simulink library "BechamoNasaOpenModels"  (R2024a)
settings: Solver=VariableStepAuto  StartTime=0.0  StopTime=10.0  RelTol=1e-3
values from neighbouring files (symbols this model uses):
  Cl_aileron_wing_1 = Cl_mat.Claileron_wing.axes1.value    [setupMavrik.m]
  Cl_aileron_wing_2 = Cl_mat.Claileron_wing.axes2.value    [setupMavrik.m]
  Cl_aileron_wing_3 = Cl_mat.Claileron_wing.axes3.value    [setupMavrik.m]
  Cl_aileron_wing_val = Cl_mat.Claileron_wing.value    [setupMavrik.m]
  Cl_elevator_tail_1 = Cl_mat.Clelevator_tail.axes1.value    [setupMavrik.m]
  Cl_elevator_tail_2 = Cl_mat.Clelevator_tail.axes2.value    [setupMavrik.m]
  Cl_elevator_tail_3 = Cl_mat.Clelevator_tail.axes3.value    [setupMavrik.m]
  Cl_elevator_tail_val = Cl_mat.Clelevator_tail.value    [setupMavrik.m]
  Cl_flap_wing_1 = Cl_mat.Clflap_wing.axes1.value    [setupMavrik.m]
  Cl_flap_wing_2 = Cl_mat.Clflap_wing.axes2.value    [setupMavrik.m]
  Cl_flap_wing_3 = Cl_mat.Clflap_wing.axes3.value    [setupMavrik.m]
  Cl_flap_wing_val = Cl_mat.Clflap_wing.value    [setupMavrik.m]
  Cl_hover_fuse_1 = Cl_mat.Clhover_fuse.axes1.value    [setupMavrik.m]
  Cl_hover_fuse_2 = Cl_mat.Clhover_fuse.axes2.value    [setupMavrik.m]
  Cl_hover_fuse_3 = Cl_mat.Clhover_fuse.axes3.value    [setupMavrik.m]
  Cl_hover_fuse_val = Cl_mat.Clhover_fuse.value    [setupMavrik.m]
  Cl_rudder_tail_1 = Cl_mat.Clrudder_tail.axes1.value    [setupMavrik.m]
  Cl_rudder_tail_2 = Cl_mat.Clrudder_tail.axes2.value    [setupMavrik.m]
  Cl_rudder_tail_3 = Cl_mat.Clrudder_tail.axes3.value    [setupMavrik.m]
  Cl_rudder_tail_val = Cl_mat.Clrudder_tail.value    [setupMavrik.m]
  Cl_tail_1 = Cl_mat.Cltail.axes1.value    [setupMavrik.m]
  Cl_tail_2 = Cl_mat.Cltail.axes2.value    [setupMavrik.m]
  Cl_tail_3 = Cl_mat.Cltail.axes3.value    [setupMavrik.m]
  Cl_tail_damp_p_1 = Cl_mat.Cltail_damp_p.axes1.value    [setupMavrik.m]
  Cl_tail_damp_p_2 = Cl_mat.Cltail_damp_p.axes2.value    [setupMavrik.m]
  Cl_tail_damp_p_3 = Cl_mat.Cltail_damp_p.axes3.value    [setupMavrik.m]
  Cl_tail_damp_p_val = Cl_mat.Cltail_damp_p.value    [setupMavrik.m]
  Cl_tail_damp_q_1 = Cl_mat.Cltail_damp_q.axes1.value    [setupMavrik.m]
  Cl_tail_damp_q_2 = Cl_mat.Cltail_damp_q.axes2.value    [setupMavrik.m]
  Cl_tail_damp_q_3 = Cl_mat.Cltail_damp_q.axes3.value    [setupMavrik.m]
  Cl_tail_damp_q_val = Cl_mat.Cltail_damp_q.value    [setupMavrik.m]
  Cl_tail_damp_r_1 = Cl_mat.Cltail_damp_r.axes1.value    [setupMavrik.m]
  Cl_tail_damp_r_2 = Cl_mat.Cltail_damp_r.axes2.value    [setupMavrik.m]
  Cl_tail_damp_r_3 = Cl_mat.Cltail_damp_r.axes3.value    [setupMavrik.m]
  Cl_tail_damp_r_val = Cl_mat.Cltail_damp_r.value    [setupMavrik.m]
  Cl_tail_val = Cl_mat.Cltail.value    [setupMavrik.m]
  Cl_wing_1 = Cl_mat.Clwing.axes1.value    [setupMavrik.m]
  Cl_wing_2 = Cl_mat.Clwing.axes2.value    [setupMavrik.m]
  Cl_wing_3 = Cl_mat.Clwing.axes3.value    [setupMavrik.m]
  Cl_wing_damp_p_1 = Cl_mat.Clwing_damp_p.axes1.value    [setupMavrik.m]
  Cl_wing_damp_p_2 = Cl_mat.Clwing_damp_p.axes2.value    [setupMavrik.m]
  Cl_wing_damp_p_3 = Cl_mat.Clwing_damp_p.axes3.value    [setupMavrik.m]
  Cl_wing_damp_p_val = Cl_mat.Clwing_damp_p.value    [setupMavrik.m]
  Cl_wing_damp_q_1 = Cl_mat.Clwing_damp_q.axes1.value    [setupMavrik.m]
  Cl_wing_damp_q_2 = Cl_mat.Clwing_damp_q.axes2.value    [setupMavrik.m]
  Cl_wing_damp_q_3 = Cl_mat.Clwing_damp_q.axes3.value    [setupMavrik.m]
  Cl_wing_damp_q_val = Cl_mat.Clwing_damp_q.value    [setupMavrik.m]
  Cl_wing_damp_r_1 = Cl_mat.Clwing_damp_r.axes1.value    [setupMavrik.m]
  Cl_wing_damp_r_2 = Cl_mat.Clwing_damp_r.axes2.value    [setupMavrik.m]
  Cl_wing_damp_r_3 = Cl_mat.Clwing_damp_r.axes3.value    [setupMavrik.m]
  Cl_wing_damp_r_val = Cl_mat.Clwing_damp_r.value    [setupMavrik.m]
  Cl_wing_val = Cl_mat.Clwing.value    [setupMavrik.m]
  Cm_aileron_wing_1 = Cm_mat.Cmaileron_wing.axes1.value    [setupMavrik.m]
  Cm_aileron_wing_2 = Cm_mat.Cmaileron_wing.axes2.value    [setupMavrik.m]
  Cm_aileron_wing_3 = Cm_mat.Cmaileron_wing.axes3.value    [setupMavrik.m]
  Cm_aileron_wing_val = Cm_mat.Cmaileron_wing.value    [setupMavrik.m]
  Cm_elevator_tail_1 = Cm_mat.Cmelevator_tail.axes1.value    [setupMavrik.m]
  Cm_elevator_tail_2 = Cm_mat.Cmelevator_tail.axes2.value    [setupMavrik.m]
  Cm_elevator_tail_3 = Cm_mat.Cmelevator_tail.axes3.value    [setupMavrik.m]
  Cm_elevator_tail_val = Cm_mat.Cmelevator_tail.value    [setupMavrik.m]
  Cm_flap_wing_1 = Cm_mat.Cmflap_wing.axes1.value    [setupMavrik.m]
  Cm_flap_wing_2 = Cm_mat.Cmflap_wing.axes2.value    [setupMavrik.m]
  Cm_flap_wing_3 = Cm_mat.Cmflap_wing.axes3.value    [setupMavrik.m]
  Cm_flap_wing_val = Cm_mat.Cmflap_wing.value    [setupMavrik.m]
  Cm_hover_fuse_1 = Cm_mat.Cmhover_fuse.axes1.value    [setupMavrik.m]
  Cm_hover_fuse_2 = Cm_mat.Cmhover_fuse.axes2.value    [setupMavrik.m]
  Cm_hover_fuse_3 = Cm_mat.Cmhover_fuse.axes3.value    [setupMavrik.m]
  Cm_hover_fuse_val = Cm_mat.Cmhover_fuse.value    [setupMavrik.m]
  Cm_rudder_tail_1 = Cm_mat.Cmrudder_tail.axes1.value    [setupMavrik.m]
  Cm_rudder_tail_2 = Cm_mat.Cmrudder_tail.axes2.value    [setupMavrik.m]
  Cm_rudder_tail_3 = Cm_mat.Cmrudder_tail.axes3.value    [setupMavrik.m]
  Cm_rudder_tail_val = Cm_mat.Cmrudder_tail.value    [setupMavrik.m]
  Cm_tail_1 = Cm_mat.Cmtail.axes1.value    [setupMavrik.m]
  Cm_tail_2 = Cm_mat.Cmtail.axes2.value    [setupMavrik.m]
  Cm_tail_3 = Cm_mat.Cmtail.axes3.value    [setupMavrik.m]
  Cm_tail_damp_p_1 = Cm_mat.Cmtail_damp_p.axes1.value    [setupMavrik.m]
  Cm_tail_damp_p_2 = Cm_mat.Cmtail_damp_p.axes2.value    [setupMavrik.m]
  Cm_tail_damp_p_3 = Cm_mat.Cmtail_damp_p.axes3.value    [setupMavrik.m]
  Cm_tail_damp_p_val = Cm_mat.Cmtail_damp_p.value    [setupMavrik.m]
  Cm_tail_damp_q_1 = Cm_mat.Cmtail_damp_q.axes1.value    [setupMavrik.m]
  Cm_tail_damp_q_2 = Cm_mat.Cmtail_damp_q.axes2.value    [setupMavrik.m]
  Cm_tail_damp_q_3 = Cm_mat.Cmtail_damp_q.axes3.value    [setupMavrik.m]
  Cm_tail_damp_q_val = Cm_mat.Cmtail_damp_q.value    [setupMavrik.m]
  Cm_tail_damp_r_1 = Cm_mat.Cmtail_damp_r.axes1.value    [setupMavrik.m]
  Cm_tail_damp_r_2 = Cm_mat.Cmtail_damp_r.axes2.value    [setupMavrik.m]
  Cm_tail_damp_r_3 = Cm_mat.Cmtail_damp_r.axes3.value    [setupMavrik.m]
  Cm_tail_damp_r_val = Cm_mat.Cmtail_damp_r.value    [setupMavrik.m]
  Cm_tail_val = Cm_mat.Cmtail.value    [setupMavrik.m]
  Cm_wing_1 = Cm_mat.Cmwing.axes1.value    [setupMavrik.m]
  Cm_wing_2 = Cm_mat.Cmwing.axes2.value    [setupMavrik.m]
  Cm_wing_3 = Cm_mat.Cmwing.axes3.value    [setupMavrik.m]
  Cm_wing_damp_p_1 = Cm_mat.Cmwing_damp_p.axes1.value    [setupMavrik.m]
  Cm_wing_damp_p_2 = Cm_mat.Cmwing_damp_p.axes2.value    [setupMavrik.m]
  Cm_wing_damp_p_3 = Cm_mat.Cmwing_damp_p.axes3.value    [setupMavrik.m]
  Cm_wing_damp_p_val = Cm_mat.Cmwing_damp_p.value    [setupMavrik.m]
  Cm_wing_damp_q_1 = Cm_mat.Cmwing_damp_q.axes1.value    [setupMavrik.m]
  Cm_wing_damp_q_2 = Cm_mat.Cmwing_damp_q.axes2.value    [setupMavrik.m]
  Cm_wing_damp_q_3 = Cm_mat.Cmwing_damp_q.axes3.value    [setupMavrik.m]
  Cm_wing_damp_q_val = Cm_mat.Cmwing_damp_q.value    [setupMavrik.m]
  Cm_wing_damp_r_1 = Cm_mat.Cmwing_damp_r.axes1.value    [setupMavrik.m]
  Cm_wing_damp_r_2 = Cm_mat.Cmwing_damp_r.axes2.value    [setupMavrik.m]
  Cm_wing_damp_r_3 = Cm_mat.Cmwing_damp_r.axes3.value    [setupMavrik.m]
  Cm_wing_damp_r_val = Cm_mat.Cmwing_damp_r.value    [setupMavrik.m]
  Cm_wing_val = Cm_mat.Cmwing.value    [setupMavrik.m]
  Cn_aileron_wing_1 = Cn_mat.Cnaileron_wing.axes1.value    [setupMavrik.m]
  Cn_aileron_wing_2 = Cn_mat.Cnaileron_wing.axes2.value    [setupMavrik.m]
  Cn_aileron_wing_3 = Cn_mat.Cnaileron_wing.axes3.value    [setupMavrik.m]
  Cn_aileron_wing_val = Cn_mat.Cnaileron_wing.value    [setupMavrik.m]
  Cn_elevator_tail_1 = Cn_mat.Cnelevator_tail.axes1.value    [setupMavrik.m]
  Cn_elevator_tail_2 = Cn_mat.Cnelevator_tail.axes2.value    [setupMavrik.m]
  Cn_elevator_tail_3 = Cn_mat.Cnelevator_tail.axes3.value    [setupMavrik.m]
  Cn_elevator_tail_val = Cn_mat.Cnelevator_tail.value    [setupMavrik.m]
  Cn_flap_wing_1 = Cn_mat.Cnflap_wing.axes1.value    [setupMavrik.m]
  Cn_flap_wing_2 = Cn_mat.Cnflap_wing.axes2.value    [setupMavrik.m]
  Cn_flap_wing_3 = Cn_mat.Cnflap_wing.axes3.value    [setupMavrik.m]
  Cn_flap_wing_val = Cn_mat.Cnflap_wing.value    [setupMavrik.m]
  Cn_hover_fuse_1 = Cn_mat.Cnhover_fuse.axes1.value    [setupMavrik.m]
  Cn_hover_fuse_2 = Cn_mat.Cnhover_fuse.axes2.value    [setupMavrik.m]
  Cn_hover_fuse_3 = Cn_mat.Cnhover_fuse.axes3.value    [setupMavrik.m]
  Cn_hover_fuse_val = Cn_mat.Cnhover_fuse.value    [setupMavrik.m]
  ... (+318 more)
libraries: matrix_library x15, shared6dof x1, sharedtransform x1
(part 3 of 19)

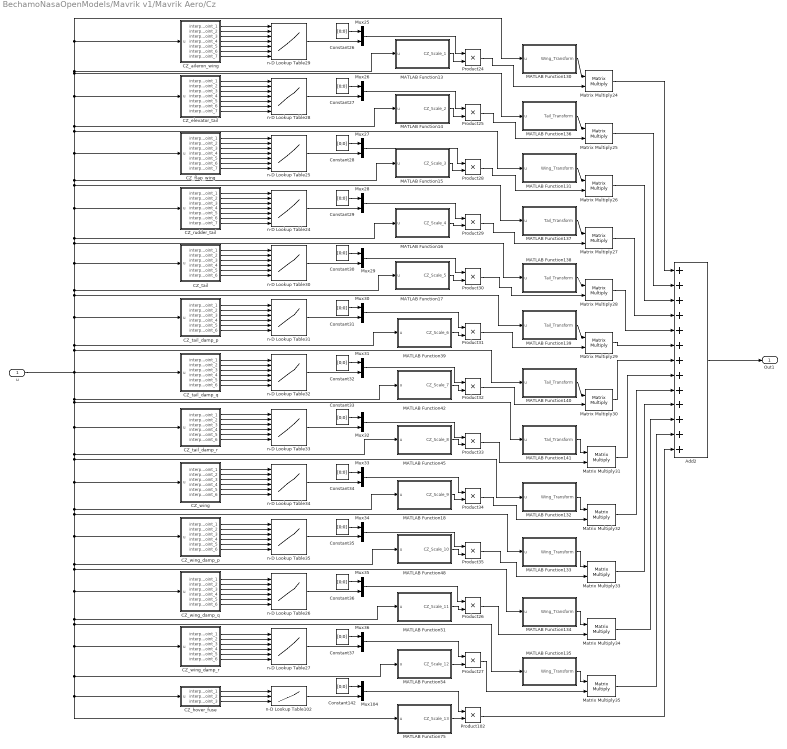
== system BechamoNasaOpenModels/Mavrik v1/Mavrik Aero/Cz ==
  u : Inport
  Add2 : Sum  Inputs=+++++++++++++
  CZ_aileron_wing : MATLAB Function  TreatAsAtomicUnit=on
  CZ_elevator_tail : MATLAB Function  TreatAsAtomicUnit=on
  CZ_flap_wing : MATLAB Function  TreatAsAtomicUnit=on
  CZ_hover_fuse : MATLAB Function  TreatAsAtomicUnit=on
  CZ_rudder_tail : MATLAB Function  TreatAsAtomicUnit=on
  CZ_tail : MATLAB Function  TreatAsAtomicUnit=on
  CZ_tail_damp_p : MATLAB Function  TreatAsAtomicUnit=on
  CZ_tail_damp_q : MATLAB Function  TreatAsAtomicUnit=on
  CZ_tail_damp_r : MATLAB Function  TreatAsAtomicUnit=on
  CZ_wing : MATLAB Function  TreatAsAtomicUnit=on
  CZ_wing_damp_p : MATLAB Function  TreatAsAtomicUnit=on
  CZ_wing_damp_q : MATLAB Function  TreatAsAtomicUnit=on
  CZ_wing_damp_r : MATLAB Function  TreatAsAtomicUnit=on
  Constant{26..37,142} (13 alike) : Constant  Value=[0;0]
  MATLAB Function13 : MATLAB Function  TreatAsAtomicUnit=on
  MATLAB Function130 : MATLAB Function  TreatAsAtomicUnit=on
  MATLAB Function131 : MATLAB Function  TreatAsAtomicUnit=on
  MATLAB Function132 : MATLAB Function  TreatAsAtomicUnit=on
  MATLAB Function133 : MATLAB Function  TreatAsAtomicUnit=on
  MATLAB Function134 : MATLAB Function  TreatAsAtomicUnit=on
  MATLAB Function135 : MATLAB Function  TreatAsAtomicUnit=on
  MATLAB Function136 : MATLAB Function  TreatAsAtomicUnit=on
  MATLAB Function137 : MATLAB Function  TreatAsAtomicUnit=on
  MATLAB Function138 : MATLAB Function  TreatAsAtomicUnit=on
  MATLAB Function139 : MATLAB Function  TreatAsAtomicUnit=on
  MATLAB Function14 : MATLAB Function  TreatAsAtomicUnit=on
  MATLAB Function140 : MATLAB Function  TreatAsAtomicUnit=on
  MATLAB Function141 : MATLAB Function  TreatAsAtomicUnit=on
  MATLAB Function15 : MATLAB Function  TreatAsAtomicUnit=on
  MATLAB Function16 : MATLAB Function  TreatAsAtomicUnit=on
  MATLAB Function17 : MATLAB Function  TreatAsAtomicUnit=on
  MATLAB Function18 : MATLAB Function  TreatAsAtomicUnit=on
  MATLAB Function39 : MATLAB Function  TreatAsAtomicUnit=on
  MATLAB Function42 : MATLAB Function  TreatAsAtomicUnit=on
  MATLAB Function45 : MATLAB Function  TreatAsAtomicUnit=on
  MATLAB Function48 : MATLAB Function  TreatAsAtomicUnit=on
  MATLAB Function51 : MATLAB Function  TreatAsAtomicUnit=on
  MATLAB Function54 : MATLAB Function  TreatAsAtomicUnit=on
  MATLAB Function75 : MATLAB Function  TreatAsAtomicUnit=on
  Matrix Multiply{24..35} (12 alike) : Product  Multiplication=Matrix(*)
  Mux{25..36,104} (13 alike) : Mux  Inputs=2
  Product{24..35,102} (13 alike) : Product
  n-D Lookup Table102 : Lookup_n-D  NumberOfTableDimensions=3  BreakpointsForDimension1=CZ_hover_fuse_1  BreakpointsForDimension2=CZ_hover_fuse_2  BreakpointsForDimension3=CZ_hover_fuse_3  BreakpointsForDimension4=CX_wing_damp_r_4  BreakpointsForDimension5=CX_wing_damp_r_5  BreakpointsForDimension6=CX_wing_damp_r_6  BreakpointsForDimension7=CX_flap_wing_7  Table=CZ_hover_fuse_val  InternalRulePriority=Speed  OutDataTypeStr=Inherit: Inherit via back propagation  RndMeth=Simplest
      settings: InputPortMap=u0,u1,u2
  n-D Lookup Table24 : Lookup_n-D  NumberOfTableDimensions=7  BreakpointsForDimension1=CZ_rudder_tail_1  BreakpointsForDimension2=CZ_rudder_tail_2  BreakpointsForDimension3=CZ_rudder_tail_3  BreakpointsForDimension4=CZ_rudder_tail_4  BreakpointsForDimension5=CZ_rudder_tail_5  BreakpointsForDimension6=CZ_rudder_tail_6  BreakpointsForDimension7=CZ_rudder_tail_7  Table=CZ_rudder_tail_val  InternalRulePriority=Speed  OutDataTypeStr=Inherit: Inherit via back propagation  RndMeth=Simplest
      settings: InputPortMap=u0,u1,u2,u3,u4,u5,u6
  n-D Lookup Table25 : Lookup_n-D  NumberOfTableDimensions=7  BreakpointsForDimension1=CZ_flap_wing_1  BreakpointsForDimension2=CZ_flap_wing_2  BreakpointsForDimension3=CZ_flap_wing_3  BreakpointsForDimension4=CZ_flap_wing_4  BreakpointsForDimension5=CZ_flap_wing_5  BreakpointsForDimension6=CZ_flap_wing_6  BreakpointsForDimension7=CZ_flap_wing_7  Table=CZ_flap_wing_val  InternalRulePriority=Speed  OutDataTypeStr=Inherit: Inherit via back propagation  RndMeth=Simplest
      settings: InputPortMap=u0,u1,u2,u3,u4,u5,u6
  n-D Lookup Table26 : Lookup_n-D  NumberOfTableDimensions=6  BreakpointsForDimension1=CZ_wing_damp_q_1  BreakpointsForDimension2=CZ_wing_damp_q_2  BreakpointsForDimension3=CZ_wing_damp_q_3  BreakpointsForDimension4=CZ_wing_damp_q_4  BreakpointsForDimension5=CZ_wing_damp_q_5  BreakpointsForDimension6=CZ_wing_damp_q_6  BreakpointsForDimension7=CX_flap_wing_7  Table=CZ_wing_damp_q_val  InternalRulePriority=Speed  OutDataTypeStr=Inherit: Inherit via back propagation  RndMeth=Simplest
      settings: InputPortMap=u0,u1,u2,u3,u4,u5
  n-D Lookup Table27 : Lookup_n-D  NumberOfTableDimensions=6  BreakpointsForDimension1=CZ_wing_damp_r_1  BreakpointsForDimension2=CZ_wing_damp_r_2  BreakpointsForDimension3=CZ_wing_damp_r_3  BreakpointsForDimension4=CZ_wing_damp_r_4  BreakpointsForDimension5=CZ_wing_damp_r_5  BreakpointsForDimension6=CZ_wing_damp_r_6  BreakpointsForDimension7=CX_flap_wing_7  Table=CZ_wing_damp_r_val  InternalRulePriority=Speed  OutDataTypeStr=Inherit: Inherit via back propagation  RndMeth=Simplest
      settings: InputPortMap=u0,u1,u2,u3,u4,u5
  n-D Lookup Table28 : Lookup_n-D  NumberOfTableDimensions=7  BreakpointsForDimension1=CZ_elevator_tail_1  BreakpointsForDimension2=CZ_elevator_tail_2  BreakpointsForDimension3=CZ_elevator_tail_3  BreakpointsForDimension4=CZ_elevator_tail_4  BreakpointsForDimension5=CZ_elevator_tail_5  BreakpointsForDimension6=CZ_elevator_tail_6  BreakpointsForDimension7=CZ_elevator_tail_7  Table=CZ_elevator_tail_val  InternalRulePriority=Speed  OutDataTypeStr=Inherit: Inherit via back propagation  RndMeth=Simplest
      settings: InputPortMap=u0,u1,u2,u3,u4,u5,u6
  n-D Lookup Table29 : Lookup_n-D  NumberOfTableDimensions=7  BreakpointsForDimension1=CZ_aileron_wing_1  BreakpointsForDimension2=CZ_aileron_wing_2  BreakpointsForDimension3=CZ_aileron_wing_3  BreakpointsForDimension4=CZ_aileron_wing_4  BreakpointsForDimension5=CZ_aileron_wing_5  BreakpointsForDimension6=CZ_aileron_wing_6  BreakpointsForDimension7=CZ_aileron_wing_7  Table=CZ_aileron_wing_val  InternalRulePriority=Speed  OutDataTypeStr=Inherit: Inherit via back propagation  RndMeth=Simplest
      settings: InputPortMap=u0,u1,u2,u3,u4,u5,u6
  n-D Lookup Table30 : Lookup_n-D  NumberOfTableDimensions=6  BreakpointsForDimension1=CZ_tail_1  BreakpointsForDimension2=CZ_tail_2  BreakpointsForDimension3=CZ_tail_3  BreakpointsForDimension4=CZ_tail_4  BreakpointsForDimension5=CZ_tail_5  BreakpointsForDimension6=CZ_tail_6  BreakpointsForDimension7=CX_tail_7  Table=CZ_tail_val  InternalRulePriority=Speed  OutDataTypeStr=Inherit: Inherit via back propagation  RndMeth=Simplest
      settings: InputPortMap=u0,u1,u2,u3,u4,u5
  n-D Lookup Table31 : Lookup_n-D  NumberOfTableDimensions=6  BreakpointsForDimension1=CZ_tail_damp_p_1  BreakpointsForDimension2=CZ_tail_damp_p_2  BreakpointsForDimension3=CZ_tail_damp_p_3  BreakpointsForDimension4=CZ_tail_damp_p_4  BreakpointsForDimension5=CZ_tail_damp_p_5  BreakpointsForDimension6=CZ_tail_damp_p_6  BreakpointsForDimension7=CX_tail_7  Table=CZ_tail_damp_p_val  InternalRulePriority=Speed  OutDataTypeStr=Inherit: Inherit via back propagation  RndMeth=Simplest
      settings: InputPortMap=u0,u1,u2,u3,u4,u5
  n-D Lookup Table32 : Lookup_n-D  NumberOfTableDimensions=6  BreakpointsForDimension1=CZ_tail_damp_q_1  BreakpointsForDimension2=CZ_tail_damp_q_2  BreakpointsForDimension3=CZ_tail_damp_q_3  BreakpointsForDimension4=CZ_tail_damp_q_4  BreakpointsForDimension5=CZ_tail_damp_q_5  BreakpointsForDimension6=CZ_tail_damp_q_6  BreakpointsForDimension7=CX_tail_7  Table=CZ_tail_damp_q_val  InternalRulePriority=Speed  OutDataTypeStr=Inherit: Inherit via back propagation  RndMeth=Simplest
      settings: InputPortMap=u0,u1,u2,u3,u4,u5
  n-D Lookup Table33 : Lookup_n-D  NumberOfTableDimensions=6  BreakpointsForDimension1=CZ_tail_damp_r_1  BreakpointsForDimension2=CZ_tail_damp_r_2  BreakpointsForDimension3=CZ_tail_damp_r_3  BreakpointsForDimension4=CZ_tail_damp_r_4  BreakpointsForDimension5=CZ_tail_damp_r_5  BreakpointsForDimension6=CZ_tail_damp_r_6  BreakpointsForDimension7=CX_tail_7  Table=CZ_tail_damp_r_val  InternalRulePriority=Speed  OutDataTypeStr=Inherit: Inherit via back propagation  RndMeth=Simplest
      settings: InputPortMap=u0,u1,u2,u3,u4,u5
  n-D Lookup Table34 : Lookup_n-D  NumberOfTableDimensions=6  BreakpointsForDimension1=CZ_wing_1  BreakpointsForDimension2=CZ_wing_2  BreakpointsForDimension3=CZ_wing_3  BreakpointsForDimension4=CZ_wing_4  BreakpointsForDimension5=CZ_wing_5  BreakpointsForDimension6=CZ_wing_6  BreakpointsForDimension7=CX_flap_wing_7  Table=CZ_wing_val  InternalRulePriority=Speed  OutDataTypeStr=Inherit: Inherit via back propagation  RndMeth=Simplest
      settings: InputPortMap=u0,u1,u2,u3,u4,u5
  n-D Lookup Table35 : Lookup_n-D  NumberOfTableDimensions=6  BreakpointsForDimension1=CZ_wing_damp_p_1  BreakpointsForDimension2=CZ_wing_damp_p_2  BreakpointsForDimension3=CZ_wing_damp_p_3  BreakpointsForDimension4=CZ_wing_damp_p_4  BreakpointsForDimension5=CZ_wing_damp_p_5  BreakpointsForDimension6=CZ_wing_damp_p_6  BreakpointsForDimension7=CX_flap_wing_7  Table=CZ_wing_damp_p_val  InternalRulePriority=Speed  OutDataTypeStr=Inherit: Inherit via back propagation  RndMeth=Simplest
      settings: InputPortMap=u0,u1,u2,u3,u4,u5
  Out1 : Outport
  wires:
  CZ_tail/2(interp_point_2) -> n-D Lookup Table30/2
  CZ_aileron_wing/2(interp_point_2) -> n-D Lookup Table29/2
  CZ_flap_wing/5(interp_point_5) -> n-D Lookup Table25/5
  Matrix Multiply27/1 -> Add2/4
  Matrix Multiply33/1 -> Add2/10
  CZ_flap_wing/3(interp_point_3) -> n-D Lookup Table25/3
  MATLAB Function18/1(CZ_Scale_9) -> Product34/2
  CZ_wing/2(interp_point_2) -> n-D Lookup Table34/2
  Matrix Multiply30/1 -> Add2/7
  MATLAB Function51/1(CZ_Scale_11) -> Product26/2
  MATLAB Function134/1(Wing_Transform) -> Matrix Multiply34/1
  Mux26/1 -> Product25/1
  Constant26/1 -> Mux25/1
  Matrix Multiply25/1 -> Add2/2
  CZ_wing_damp_q/1(interp_point_1) -> n-D Lookup Table26/1
  Matrix Multiply26/1 -> Add2/3
  Mux28/1 -> Product29/1
  Matrix Multiply35/1 -> Add2/12
  CZ_rudder_tail/7(interp_point_7) -> n-D Lookup Table24/7
  CZ_wing_damp_r/4(interp_point_4) -> n-D Lookup Table27/4
  CZ_wing_damp_q/5(interp_point_5) -> n-D Lookup Table26/5
  Mux104/1 -> Product102/1
  CZ_wing_damp_p/6(interp_point_6) -> n-D Lookup Table35/6
  CZ_elevator_tail/3(interp_point_3) -> n-D Lookup Table28/3
  n-D Lookup Table27/1 -> Mux36/2
  CZ_wing_damp_r/1(interp_point_1) -> n-D Lookup Table27/1
  CZ_tail_damp_q/3(interp_point_3) -> n-D Lookup Table32/3
  CZ_tail_damp_r/3(interp_point_3) -> n-D Lookup Table33/3
  Matrix Multiply32/1 -> Add2/9
  Mux31/1 -> Product32/1
  CZ_flap_wing/4(interp_point_4) -> n-D Lookup Table25/4
  CZ_flap_wing/1(interp_point_1) -> n-D Lookup Table25/1
  Mux35/1 -> Product26/1
  Matrix Multiply29/1 -> Add2/6
  Mux34/1 -> Product35/1
  Mux29/1 -> Product30/1
  Mux25/1 -> Product24/1
  CZ_tail_damp_p/1(interp_point_1) -> n-D Lookup Table31/1
  CZ_elevator_tail/5(interp_point_5) -> n-D Lookup Table28/5
  Product32/1 -> Matrix Multiply30/2
  CZ_tail/4(interp_point_4) -> n-D Lookup Table30/4
  Constant35/1 -> Mux34/1
  CZ_flap_wing/7(interp_point_7) -> n-D Lookup Table25/7
  n-D Lookup Table33/1 -> Mux32/2
  CZ_wing_damp_r/2(interp_point_2) -> n-D Lookup Table27/2
  CZ_tail_damp_r/1(interp_point_1) -> n-D Lookup Table33/1
  CZ_wing_damp_p/2(interp_point_2) -> n-D Lookup Table35/2
  MATLAB Function13/1(CZ_Scale_1) -> Product24/2
  Constant32/1 -> Mux31/1
  MATLAB Function138/1(Tail_Transform) -> Matrix Multiply28/1
  CZ_tail_damp_r/5(interp_point_5) -> n-D Lookup Table33/5
  CZ_aileron_wing/7(interp_point_7) -> n-D Lookup Table29/7
  CZ_tail_damp_p/6(interp_point_6) -> n-D Lookup Table31/6
  Product34/1 -> Matrix Multiply32/2
  CZ_tail_damp_r/4(interp_point_4) -> n-D Lookup Table33/4
  CZ_wing_damp_r/3(interp_point_3) -> n-D Lookup Table27/3
  CZ_tail_damp_q/5(interp_point_5) -> n-D Lookup Table32/5
  CZ_elevator_tail/6(interp_point_6) -> n-D Lookup Table28/6
  MATLAB Function132/1(Wing_Transform) -> Matrix Multiply32/1
  n-D Lookup Table30/1 -> Mux29/2
  CZ_rudder_tail/4(interp_point_4) -> n-D Lookup Table24/4
  CZ_flap_wing/6(interp_point_6) -> n-D Lookup Table25/6
  Mux27/1 -> Product28/1
  Mux30/1 -> Product31/1
  CZ_wing/4(interp_point_4) -> n-D Lookup Table34/4
  CZ_tail_damp_p/4(interp_point_4) -> n-D Lookup Table31/4
  CZ_elevator_tail/7(interp_point_7) -> n-D Lookup Table28/7
  n-D Lookup Table28/1 -> Mux26/2
  Constant31/1 -> Mux30/1
  CZ_tail_damp_p/2(interp_point_2) -> n-D Lookup Table31/2
  CZ_aileron_wing/6(interp_point_6) -> n-D Lookup Table29/6
  CZ_rudder_tail/1(interp_point_1) -> n-D Lookup Table24/1
  MATLAB Function137/1(Tail_Transform) -> Matrix Multiply27/1
  CZ_tail_damp_q/1(interp_point_1) -> n-D Lookup Table32/1
  CZ_tail_damp_p/3(interp_point_3) -> n-D Lookup Table31/3
  CZ_wing_damp_p/3(interp_point_3) -> n-D Lookup Table35/3
  CZ_elevator_tail/1(interp_point_1) -> n-D Lookup Table28/1
  CZ_wing/3(interp_point_3) -> n-D Lookup Table34/3
  CZ_tail/6(interp_point_6) -> n-D Lookup Table30/6
  CZ_wing_damp_p/4(interp_point_4) -> n-D Lookup Table35/4
  CZ_wing_damp_q/6(interp_point_6) -> n-D Lookup Table26/6
  CZ_wing/5(interp_point_5) -> n-D Lookup Table34/5
  CZ_wing_damp_r/6(interp_point_6) -> n-D Lookup Table27/6
  MATLAB Function75/1(CZ_Scale_13) -> Product102/2
  CZ_tail/1(interp_point_1) -> n-D Lookup Table30/1
  Mux33/1 -> Product34/1
  CZ_aileron_wing/3(interp_point_3) -> n-D Lookup Table29/3
  CZ_tail_damp_r/2(interp_point_2) -> n-D Lookup Table33/2
  MATLAB Function17/1(CZ_Scale_5) -> Product30/2
  MATLAB Function133/1(Wing_Transform) -> Matrix Multiply33/1
  Matrix Multiply24/1 -> Add2/1
  CZ_aileron_wing/4(interp_point_4) -> n-D Lookup Table29/4
  MATLAB Function131/1(Wing_Transform) -> Matrix Multiply26/1
  Product30/1 -> Matrix Multiply28/2
  CZ_tail/3(interp_point_3) -> n-D Lookup Table30/3
  CZ_flap_wing/2(interp_point_2) -> n-D Lookup Table25/2
  CZ_aileron_wing/5(interp_point_5) -> n-D Lookup Table29/5
  n-D Lookup Table34/1 -> Mux33/2
  n-D Lookup Table35/1 -> Mux34/2
  MATLAB Function135/1(Wing_Transform) -> Matrix Multiply35/1
  Constant36/1 -> Mux35/1
  Product25/1 -> Matrix Multiply25/2
  Constant33/1 -> Mux32/1
  MATLAB Function136/1(Tail_Transform) -> Matrix Multiply25/1
  CZ_wing_damp_p/5(interp_point_5) -> n-D Lookup Table35/5
  MATLAB Function139/1(Tail_Transform) -> Matrix Multiply29/1
  CZ_tail/5(interp_point_5) -> n-D Lookup Table30/5
  MATLAB Function45/1(CZ_Scale_8) -> Product33/2
  MATLAB Function140/1(Tail_Transform) -> Matrix Multiply30/1
  Product102/1 -> Add2/13
  n-D Lookup Table31/1 -> Mux30/2
  CZ_hover_fuse/2(interp_point_2) -> n-D Lookup Table102/2
  CZ_elevator_tail/2(interp_point_2) -> n-D Lookup Table28/2
  CZ_rudder_tail/2(interp_point_2) -> n-D Lookup Table24/2
  CZ_hover_fuse/1(interp_point_1) -> n-D Lookup Table102/1
  CZ_hover_fuse/3(interp_point_3) -> n-D Lookup Table102/3
  Matrix Multiply34/1 -> Add2/11
  Product35/1 -> Matrix Multiply33/2
  Matrix Multiply28/1 -> Add2/5
  Matrix Multiply31/1 -> Add2/8
  Mux36/1 -> Product27/1
  MATLAB Function141/1(Tail_Transform) -> Matrix Multiply31/1
  CZ_wing_damp_q/4(interp_point_4) -> n-D Lookup Table26/4
  Constant27/1 -> Mux26/1
  Constant34/1 -> Mux33/1
  n-D Lookup Table25/1 -> Mux27/2
  CZ_tail_damp_q/2(interp_point_2) -> n-D Lookup Table32/2
  Constant29/1 -> Mux28/1
  n-D Lookup Table26/1 -> Mux35/2
  Constant37/1 -> Mux36/1
  Product28/1 -> Matrix Multiply26/2
  CZ_wing/1(interp_point_1) -> n-D Lookup Table34/1
  Constant30/1 -> Mux29/1
  CZ_wing/6(interp_point_6) -> n-D Lookup Table34/6
  CZ_rudder_tail/5(interp_point_5) -> n-D Lookup Table24/5
  MATLAB Function54/1(CZ_Scale_12) -> Product27/2
  Constant28/1 -> Mux27/1
  Product26/1 -> Matrix Multiply34/2
  MATLAB Function130/1(Wing_Transform) -> Matrix Multiply24/1
  CZ_tail_damp_q/4(interp_point_4) -> n-D Lookup Table32/4
  Product29/1 -> Matrix Multiply27/2
  CZ_wing_damp_r/5(interp_point_5) -> n-D Lookup Table27/5
  Mux32/1 -> Product33/1
  Product33/1 -> Matrix Multiply31/2
  n-D Lookup Table29/1 -> Mux25/2
  Product27/1 -> Matrix Multiply35/2
  CZ_elevator_tail/4(interp_point_4) -> n-D Lookup Table28/4
  CZ_rudder_tail/3(interp_point_3) -> n-D Lookup Table24/3
  MATLAB Function14/1(CZ_Scale_2) -> Product25/2
  CZ_wing_damp_q/2(interp_point_2) -> n-D Lookup Table26/2
  MATLAB Function42/1(CZ_Scale_7) -> Product32/2
  CZ_tail_damp_p/5(interp_point_5) -> n-D Lookup Table31/5
  MATLAB Function48/1(CZ_Scale_10) -> Product35/2
  MATLAB Function39/1(CZ_Scale_6) -> Product31/2
  CZ_aileron_wing/1(interp_point_1) -> n-D Lookup Table29/1
  CZ_tail_damp_q/6(interp_point_6) -> n-D Lookup Table32/6
  n-D Lookup Table32/1 -> Mux31/2
  n-D Lookup Table102/1 -> Mux104/2
  Constant142/1 -> Mux104/1
  CZ_rudder_tail/6(interp_point_6) -> n-D Lookup Table24/6
  Product31/1 -> Matrix Multiply29/2
  MATLAB Function16/1(CZ_Scale_4) -> Product29/2
  MATLAB Function15/1(CZ_Scale_3) -> Product28/2
  Product24/1 -> Matrix Multiply24/2
  CZ_wing_damp_p/1(interp_point_1) -> n-D Lookup Table35/1
  CZ_wing_damp_q/3(interp_point_3) -> n-D Lookup Table26/3
  CZ_tail_damp_r/6(interp_point_6) -> n-D Lookup Table33/6
  n-D Lookup Table24/1 -> Mux28/2
  Add2/1 -> Out1/1
  u/1 -> MATLAB Function42/1(u), MATLAB Function141/1(u), CZ_tail_damp_r/1(u), MATLAB Function45/1(u), MATLAB Function132/1(u), CZ_wing/1(u), MATLAB Function18/1(u), MATLAB Function133/1(u), CZ_wing_damp_p/1(u), MATLAB Function48/1(u), MATLAB Function134/1(u), CZ_wing_damp_q/1(u), MATLAB Function51/1(u), MATLAB Function135/1(u), CZ_wing_damp_r/1(u), MATLAB Function54/1(u), CZ_hover_fuse/1(u), MATLAB Function75/1(u), MATLAB Function140/1(u), MATLAB Function39/1(u), CZ_tail_damp_p/1(u), MATLAB Function139/1(u), MATLAB Function17/1(u), CZ_tail/1(u), MATLAB Function138/1(u), MATLAB Function16/1(u), MATLAB Function137/1(u), CZ_flap_wing/1(u), MATLAB Function131/1(u), CZ_elevator_tail/1(u), MATLAB Function136/1(u), MATLAB Function13/1(u), CZ_aileron_wing/1(u), MATLAB Function130/1(u), MATLAB Function14/1(u), MATLAB Function15/1(u), CZ_rudder_tail/1(u), CZ_tail_damp_q/1(u)

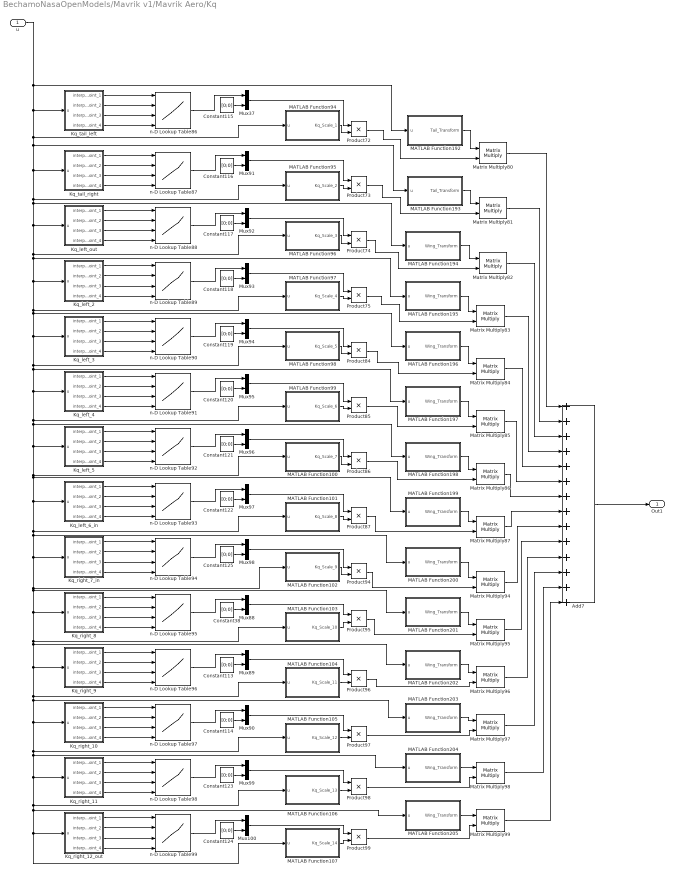
== system BechamoNasaOpenModels/Mavrik v1/Mavrik Aero/Kq ==
  u : Inport
  Add7 : Sum  Inputs=++++++++++++++
  Constant{38,113..125} (14 alike) : Constant  Value=[0;0]
  Kq_left_2 : MATLAB Function  TreatAsAtomicUnit=on
  Kq_left_3 : MATLAB Function  TreatAsAtomicUnit=on
  Kq_left_4 : MATLAB Function  TreatAsAtomicUnit=on
  Kq_left_5 : MATLAB Function  TreatAsAtomicUnit=on
  Kq_left_6_in : MATLAB Function  TreatAsAtomicUnit=on
  Kq_left_out : MATLAB Function  TreatAsAtomicUnit=on
  Kq_right_10 : MATLAB Function  TreatAsAtomicUnit=on
  Kq_right_11 : MATLAB Function  TreatAsAtomicUnit=on
  Kq_right_12_out : MATLAB Function  TreatAsAtomicUnit=on
  Kq_right_7_in : MATLAB Function  TreatAsAtomicUnit=on
  Kq_right_8 : MATLAB Function  TreatAsAtomicUnit=on
  Kq_right_9 : MATLAB Function  TreatAsAtomicUnit=on
  Kq_tail_left : MATLAB Function  TreatAsAtomicUnit=on
  Kq_tail_right : MATLAB Function  TreatAsAtomicUnit=on
  MATLAB Function100 : MATLAB Function  TreatAsAtomicUnit=on
  MATLAB Function101 : MATLAB Function  TreatAsAtomicUnit=on
  MATLAB Function102 : MATLAB Function  TreatAsAtomicUnit=on
  MATLAB Function103 : MATLAB Function  TreatAsAtomicUnit=on
  MATLAB Function104 : MATLAB Function  TreatAsAtomicUnit=on
  MATLAB Function105 : MATLAB Function  TreatAsAtomicUnit=on
  MATLAB Function106 : MATLAB Function  TreatAsAtomicUnit=on
  MATLAB Function107 : MATLAB Function  TreatAsAtomicUnit=on
  MATLAB Function192 : MATLAB Function  TreatAsAtomicUnit=on
  MATLAB Function193 : MATLAB Function  TreatAsAtomicUnit=on
  MATLAB Function194 : MATLAB Function  TreatAsAtomicUnit=on
  MATLAB Function195 : MATLAB Function  TreatAsAtomicUnit=on
  MATLAB Function196 : MATLAB Function  TreatAsAtomicUnit=on
  MATLAB Function197 : MATLAB Function  TreatAsAtomicUnit=on
  MATLAB Function198 : MATLAB Function  TreatAsAtomicUnit=on
  MATLAB Function199 : MATLAB Function  TreatAsAtomicUnit=on
  MATLAB Function200 : MATLAB Function  TreatAsAtomicUnit=on
  MATLAB Function201 : MATLAB Function  TreatAsAtomicUnit=on
  MATLAB Function202 : MATLAB Function  TreatAsAtomicUnit=on
  MATLAB Function203 : MATLAB Function  TreatAsAtomicUnit=on
  MATLAB Function204 : MATLAB Function  TreatAsAtomicUnit=on
  MATLAB Function205 : MATLAB Function  TreatAsAtomicUnit=on
  MATLAB Function94 : MATLAB Function  TreatAsAtomicUnit=on
  MATLAB Function95 : MATLAB Function  TreatAsAtomicUnit=on
  MATLAB Function96 : MATLAB Function  TreatAsAtomicUnit=on
  MATLAB Function97 : MATLAB Function  TreatAsAtomicUnit=on
  MATLAB Function98 : MATLAB Function  TreatAsAtomicUnit=on
  MATLAB Function99 : MATLAB Function  TreatAsAtomicUnit=on
  Matrix Multiply{80..87,94..99} (14 alike) : Product  Multiplication=Matrix(*)
  Mux{37,88..100} (14 alike) : Mux  Inputs=2
  Product{72..75,84..87,94..99} (14 alike) : Product
  n-D Lookup Table86 : Lookup_n-D  NumberOfTableDimensions=4  BreakpointsForDimension1=Kq_tail_left_1  BreakpointsForDimension2=Kq_tail_left_2  BreakpointsForDimension3=Kq_tail_left_3  BreakpointsForDimension4=Kq_tail_left_4  BreakpointsForDimension5=Cn_wing_damp_r_5  BreakpointsForDimension6=Cn_wing_damp_r_6  BreakpointsForDimension7=CX_flap_wing_7  Table=Kq_tail_left_val  InternalRulePriority=Speed  OutDataTypeStr=Inherit: Inherit via back propagation  RndMeth=Simplest
      settings: InputPortMap=u0,u1,u2,u3
  n-D Lookup Table87 : Lookup_n-D  NumberOfTableDimensions=4  BreakpointsForDimension1=Kq_tail_right_1  BreakpointsForDimension2=Kq_tail_right_2  BreakpointsForDimension3=Kq_tail_right_3  BreakpointsForDimension4=Kq_tail_right_4  BreakpointsForDimension5=Cn_wing_damp_r_5  BreakpointsForDimension6=Cn_wing_damp_r_6  BreakpointsForDimension7=CX_flap_wing_7  Table=Kq_tail_right_val  InternalRulePriority=Speed  OutDataTypeStr=Inherit: Inherit via back propagation  RndMeth=Simplest
      settings: InputPortMap=u0,u1,u2,u3
  n-D Lookup Table88 : Lookup_n-D  NumberOfTableDimensions=4  BreakpointsForDimension1=Kq_left_out_1  BreakpointsForDimension2=Kq_left_out_2  BreakpointsForDimension3=Kq_left_out_3  BreakpointsForDimension4=Kq_left_out_4  BreakpointsForDimension5=Cn_wing_damp_r_5  BreakpointsForDimension6=Cn_wing_damp_r_6  BreakpointsForDimension7=CX_flap_wing_7  Table=Kq_left_out_val  InternalRulePriority=Speed  OutDataTypeStr=Inherit: Inherit via back propagation  RndMeth=Simplest
      settings: InputPortMap=u0,u1,u2,u3
  n-D Lookup Table89 : Lookup_n-D  NumberOfTableDimensions=4  BreakpointsForDimension1=Kq_left_2_1  BreakpointsForDimension2=Kq_left_2_2  BreakpointsForDimension3=Kq_left_2_3  BreakpointsForDimension4=Kq_left_2_4  BreakpointsForDimension5=Cn_wing_damp_r_5  BreakpointsForDimension6=Cn_wing_damp_r_6  BreakpointsForDimension7=CX_flap_wing_7  Table=Kq_left_2_val  InternalRulePriority=Speed  OutDataTypeStr=Inherit: Inherit via back propagation  RndMeth=Simplest
      settings: InputPortMap=u0,u1,u2,u3
  n-D Lookup Table90 : Lookup_n-D  NumberOfTableDimensions=4  BreakpointsForDimension1=Kq_left_3_1  BreakpointsForDimension2=Kq_left_3_2  BreakpointsForDimension3=Kq_left_3_3  BreakpointsForDimension4=Kq_left_3_4  BreakpointsForDimension5=Cn_wing_damp_r_5  BreakpointsForDimension6=Cn_wing_damp_r_6  BreakpointsForDimension7=CX_flap_wing_7  Table=Kq_left_3_val  InternalRulePriority=Speed  OutDataTypeStr=Inherit: Inherit via back propagation  RndMeth=Simplest
      settings: InputPortMap=u0,u1,u2,u3
  n-D Lookup Table91 : Lookup_n-D  NumberOfTableDimensions=4  BreakpointsForDimension1=Kq_left_4_1  BreakpointsForDimension2=Kq_left_4_2  BreakpointsForDimension3=Kq_left_4_3  BreakpointsForDimension4=Kq_left_4_4  BreakpointsForDimension5=Cn_wing_damp_r_5  BreakpointsForDimension6=Cn_wing_damp_r_6  BreakpointsForDimension7=CX_flap_wing_7  Table=Kq_left_4_val  InternalRulePriority=Speed  OutDataTypeStr=Inherit: Inherit via back propagation  RndMeth=Simplest
      settings: InputPortMap=u0,u1,u2,u3
  n-D Lookup Table92 : Lookup_n-D  NumberOfTableDimensions=4  BreakpointsForDimension1=Kq_left_5_1  BreakpointsForDimension2=Kq_left_5_2  BreakpointsForDimension3=Kq_left_5_3  BreakpointsForDimension4=Kq_left_5_4  BreakpointsForDimension5=Cn_wing_damp_r_5  BreakpointsForDimension6=Cn_wing_damp_r_6  BreakpointsForDimension7=CX_flap_wing_7  Table=Kq_left_5_val  InternalRulePriority=Speed  OutDataTypeStr=Inherit: Inherit via back propagation  RndMeth=Simplest
      settings: InputPortMap=u0,u1,u2,u3
  n-D Lookup Table93 : Lookup_n-D  NumberOfTableDimensions=4  BreakpointsForDimension1=Kq_left_6_in_1  BreakpointsForDimension2=Kq_left_6_in_2  BreakpointsForDimension3=Kq_left_6_in_3  BreakpointsForDimension4=Kq_left_6_in_4  BreakpointsForDimension5=Cn_wing_damp_r_5  BreakpointsForDimension6=Cn_wing_damp_r_6  BreakpointsForDimension7=CX_flap_wing_7  Table=Kq_left_6_in_val  InternalRulePriority=Speed  OutDataTypeStr=Inherit: Inherit via back propagation  RndMeth=Simplest
      settings: InputPortMap=u0,u1,u2,u3
  n-D Lookup Table94 : Lookup_n-D  NumberOfTableDimensions=4  BreakpointsForDimension1=Kq_right_7_in_1  BreakpointsForDimension2=Kq_right_7_in_2  BreakpointsForDimension3=Kq_right_7_in_3  BreakpointsForDimension4=Kq_right_7_in_4  BreakpointsForDimension5=Cn_wing_damp_r_5  BreakpointsForDimension6=Cn_wing_damp_r_6  BreakpointsForDimension7=CX_flap_wing_7  Table=Kq_right_7_in_val  InternalRulePriority=Speed  OutDataTypeStr=Inherit: Inherit via back propagation  RndMeth=Simplest
      settings: InputPortMap=u0,u1,u2,u3
  n-D Lookup Table95 : Lookup_n-D  NumberOfTableDimensions=4  BreakpointsForDimension1=Kq_right_8_1  BreakpointsForDimension2=Kq_right_8_2  BreakpointsForDimension3=Kq_right_8_3  BreakpointsForDimension4=Kq_right_8_4  BreakpointsForDimension5=Cn_wing_damp_r_5  BreakpointsForDimension6=Cn_wing_damp_r_6  BreakpointsForDimension7=CX_flap_wing_7  Table=Kq_right_8_val  InternalRulePriority=Speed  OutDataTypeStr=Inherit: Inherit via back propagation  RndMeth=Simplest
      settings: InputPortMap=u0,u1,u2,u3
  n-D Lookup Table96 : Lookup_n-D  NumberOfTableDimensions=4  BreakpointsForDimension1=Kq_right_9_1  BreakpointsForDimension2=Kq_right_9_2  BreakpointsForDimension3=Kq_right_9_3  BreakpointsForDimension4=Kq_right_9_4  BreakpointsForDimension5=Cn_wing_damp_r_5  BreakpointsForDimension6=Cn_wing_damp_r_6  BreakpointsForDimension7=CX_flap_wing_7  Table=Kq_right_9_val  InternalRulePriority=Speed  OutDataTypeStr=Inherit: Inherit via back propagation  RndMeth=Simplest
      settings: InputPortMap=u0,u1,u2,u3
  n-D Lookup Table97 : Lookup_n-D  NumberOfTableDimensions=4  BreakpointsForDimension1=Kq_right_10_1  BreakpointsForDimension2=Kq_right_10_2  BreakpointsForDimension3=Kq_right_10_3  BreakpointsForDimension4=Kq_right_10_4  BreakpointsForDimension5=Cn_wing_damp_r_5  BreakpointsForDimension6=Cn_wing_damp_r_6  BreakpointsForDimension7=CX_flap_wing_7  Table=Kq_right_10_val  InternalRulePriority=Speed  OutDataTypeStr=Inherit: Inherit via back propagation  RndMeth=Simplest
      settings: InputPortMap=u0,u1,u2,u3
  n-D Lookup Table98 : Lookup_n-D  NumberOfTableDimensions=4  BreakpointsForDimension1=Kq_right_11_1  BreakpointsForDimension2=Kq_right_11_2  BreakpointsForDimension3=Kq_right_11_3  BreakpointsForDimension4=Kq_right_11_4  BreakpointsForDimension5=Cn_wing_damp_r_5  BreakpointsForDimension6=Cn_wing_damp_r_6  BreakpointsForDimension7=CX_flap_wing_7  Table=Kq_right_11_val  InternalRulePriority=Speed  OutDataTypeStr=Inherit: Inherit via back propagation  RndMeth=Simplest
      settings: InputPortMap=u0,u1,u2,u3
  n-D Lookup Table99 : Lookup_n-D  NumberOfTableDimensions=4  BreakpointsForDimension1=Kq_right_12_out_1  BreakpointsForDimension2=Kq_right_12_out_2  BreakpointsForDimension3=Kq_right_12_out_3  BreakpointsForDimension4=Kq_right_12_out_4  BreakpointsForDimension5=Cn_wing_damp_r_5  BreakpointsForDimension6=Cn_wing_damp_r_6  BreakpointsForDimension7=CX_flap_wing_7  Table=Kq_right_12_out_val  InternalRulePriority=Speed  OutDataTypeStr=Inherit: Inherit via back propagation  RndMeth=Simplest
      settings: InputPortMap=u0,u1,u2,u3
  Out1 : Outport
  wires:
  Mux92/1 -> Product74/1
  MATLAB Function101/1(Kq_Scale_8) -> Product87/2
  Mux91/1 -> Product73/1
  Mux95/1 -> Product85/1
  Mux88/1 -> Product95/1
  Kq_right_9/3(interp_point_3) -> n-D Lookup Table96/3
  Mux94/1 -> Product84/1
  Kq_left_3/4(interp_point_4) -> n-D Lookup Table90/4
  MATLAB Function205/1(Wing_Transform) -> Matrix Multiply99/1
  Kq_tail_right/4(interp_point_4) -> n-D Lookup Table87/4
  Mux96/1 -> Product86/1
  Kq_left_out/1(interp_point_1) -> n-D Lookup Table88/1
  Constant122/1 -> Mux97/2
  n-D Lookup Table92/1 -> Mux96/1
  MATLAB Function201/1(Wing_Transform) -> Matrix Multiply95/1
  u/1 -> MATLAB Function192/1(u), Kq_tail_left/1(u), MATLAB Function94/1(u), MATLAB Function193/1(u), Kq_tail_right/1(u), MATLAB Function95/1(u), MATLAB Function194/1(u), Kq_left_out/1(u), MATLAB Function96/1(u), MATLAB Function195/1(u), Kq_left_2/1(u), MATLAB Function97/1(u), Kq_left_3/1(u), MATLAB Function98/1(u), MATLAB Function197/1(u), Kq_left_4/1(u), MATLAB Function99/1(u), MATLAB Function198/1(u), Kq_left_5/1(u), MATLAB Function100/1(u), MATLAB Function199/1(u), Kq_left_6_in/1(u), MATLAB Function101/1(u), MATLAB Function200/1(u), Kq_right_7_in/1(u), MATLAB Function102/1(u), MATLAB Function201/1(u), Kq_right_8/1(u), MATLAB Function103/1(u), Kq_right_9/1(u), MATLAB Function104/1(u), MATLAB Function203/1(u), Kq_right_10/1(u), MATLAB Function105/1(u), Kq_right_11/1(u), MATLAB Function106/1(u), MATLAB Function205/1(u), Kq_right_12_out/1(u), MATLAB Function107/1(u), MATLAB Function204/1(u), MATLAB Function202/1(u), MATLAB Function196/1(u)
  Product74/1 -> Matrix Multiply82/2
  Kq_left_6_in/3(interp_point_3) -> n-D Lookup Table93/3
  MATLAB Function97/1(Kq_Scale_4) -> Product75/2
  Product99/1 -> Matrix Multiply99/2
  Kq_right_10/1(interp_point_1) -> n-D Lookup Table97/1
  Matrix Multiply87/1 -> Add7/8
  Matrix Multiply86/1 -> Add7/7
  Mux93/1 -> Product75/1
  Product85/1 -> Matrix Multiply85/2
  n-D Lookup Table99/1 -> Mux100/1
  Constant119/1 -> Mux94/2
  MATLAB Function103/1(Kq_Scale_10) -> Product95/2
  Kq_left_4/3(interp_point_3) -> n-D Lookup Table91/3
  MATLAB Function105/1(Kq_Scale_12) -> Product97/2
  Matrix Multiply81/1 -> Add7/2
  Kq_left_5/4(interp_point_4) -> n-D Lookup Table92/4
  n-D Lookup Table87/1 -> Mux91/1
  Kq_tail_right/1(interp_point_1) -> n-D Lookup Table87/1
  Kq_right_10/4(interp_point_4) -> n-D Lookup Table97/4
  Kq_left_2/4(interp_point_4) -> n-D Lookup Table89/4
  Constant116/1 -> Mux91/2
  Constant120/1 -> Mux95/2
  MATLAB Function193/1(Tail_Transform) -> Matrix Multiply81/1
  MATLAB Function95/1(Kq_Scale_2) -> Product73/2
  n-D Lookup Table86/1 -> Mux37/1
  Kq_left_3/1(interp_point_1) -> n-D Lookup Table90/1
  Product96/1 -> Matrix Multiply96/2
  Kq_left_5/2(interp_point_2) -> n-D Lookup Table92/2
  MATLAB Function107/1(Kq_Scale_14) -> Product99/2
  n-D Lookup Table98/1 -> Mux99/1
  Mux37/1 -> Product72/1
  MATLAB Function99/1(Kq_Scale_6) -> Product85/2
  Constant118/1 -> Mux93/2
  Product73/1 -> Matrix Multiply81/2
  Mux89/1 -> Product96/1
  Constant114/1 -> Mux90/2
  Kq_tail_left/4(interp_point_4) -> n-D Lookup Table86/4
  n-D Lookup Table90/1 -> Mux94/1
  Product94/1 -> Matrix Multiply94/2
  Constant115/1 -> Mux37/2
  n-D Lookup Table96/1 -> Mux89/1
  Mux98/1 -> Product94/1
  n-D Lookup Table94/1 -> Mux98/1
  Matrix Multiply98/1 -> Add7/13
  MATLAB Function100/1(Kq_Scale_7) -> Product86/2
  Constant123/1 -> Mux99/2
  Kq_right_10/2(interp_point_2) -> n-D Lookup Table97/2
  MATLAB Function94/1(Kq_Scale_1) -> Product72/2
  Kq_right_8/1(interp_point_1) -> n-D Lookup Table95/1
  Constant113/1 -> Mux89/2
  n-D Lookup Table88/1 -> Mux92/1
  Constant125/1 -> Mux98/2
  Kq_right_12_out/2(interp_point_2) -> n-D Lookup Table99/2
  Kq_left_out/2(interp_point_2) -> n-D Lookup Table88/2
  Product75/1 -> Matrix Multiply83/2
  n-D Lookup Table91/1 -> Mux95/1
  Kq_right_7_in/2(interp_point_2) -> n-D Lookup Table94/2
  Kq_right_11/2(interp_point_2) -> n-D Lookup Table98/2
  Product84/1 -> Matrix Multiply84/2
  Kq_right_11/4(interp_point_4) -> n-D Lookup Table98/4
  Matrix Multiply80/1 -> Add7/1
  Matrix Multiply82/1 -> Add7/3
  Kq_right_11/3(interp_point_3) -> n-D Lookup Table98/3
  MATLAB Function106/1(Kq_Scale_13) -> Product98/2
  Product72/1 -> Matrix Multiply80/2
  MATLAB Function195/1(Wing_Transform) -> Matrix Multiply83/1
  Kq_tail_left/2(interp_point_2) -> n-D Lookup Table86/2
  Mux97/1 -> Product87/1
  MATLAB Function204/1(Wing_Transform) -> Matrix Multiply98/1
  Matrix Multiply85/1 -> Add7/6
  Kq_left_4/4(interp_point_4) -> n-D Lookup Table91/4
  Kq_right_9/2(interp_point_2) -> n-D Lookup Table96/2
  Matrix Multiply94/1 -> Add7/9
  Kq_left_2/2(interp_point_2) -> n-D Lookup Table89/2
  Product97/1 -> Matrix Multiply97/2
  Matrix Multiply96/1 -> Add7/11
  Constant38/1 -> Mux88/2
  Product98/1 -> Matrix Multiply98/2
  Matrix Multiply99/1 -> Add7/14
  Matrix Multiply97/1 -> Add7/12
  Mux100/1 -> Product99/1
  Product86/1 -> Matrix Multiply86/2
  Kq_right_7_in/1(interp_point_1) -> n-D Lookup Table94/1
  Kq_left_4/1(interp_point_1) -> n-D Lookup Table91/1
  Kq_right_7_in/4(interp_point_4) -> n-D Lookup Table94/4
  Kq_right_11/1(interp_point_1) -> n-D Lookup Table98/1
  Kq_right_7_in/3(interp_point_3) -> n-D Lookup Table94/3
  Kq_left_5/3(interp_point_3) -> n-D Lookup Table92/3
  Kq_tail_right/3(interp_point_3) -> n-D Lookup Table87/3
  Kq_right_12_out/3(interp_point_3) -> n-D Lookup Table99/3
  Kq_right_8/2(interp_point_2) -> n-D Lookup Table95/2
  Kq_left_6_in/2(interp_point_2) -> n-D Lookup Table93/2
  Kq_tail_left/1(interp_point_1) -> n-D Lookup Table86/1
  Kq_left_2/1(interp_point_1) -> n-D Lookup Table89/1
  n-D Lookup Table89/1 -> Mux93/1
  MATLAB Function104/1(Kq_Scale_11) -> Product96/2
  Kq_left_4/2(interp_point_2) -> n-D Lookup Table91/2
  Product87/1 -> Matrix Multiply87/2
  Kq_right_9/1(interp_point_1) -> n-D Lookup Table96/1
  Kq_tail_left/3(interp_point_3) -> n-D Lookup Table86/3
  Kq_left_3/3(interp_point_3) -> n-D Lookup Table90/3
  Matrix Multiply83/1 -> Add7/4
  Kq_right_12_out/4(interp_point_4) -> n-D Lookup Table99/4
  Kq_left_3/2(interp_point_2) -> n-D Lookup Table90/2
  Kq_left_5/1(interp_point_1) -> n-D Lookup Table92/1
  Kq_right_8/3(interp_point_3) -> n-D Lookup Table95/3
  Kq_left_2/3(interp_point_3) -> n-D Lookup Table89/3
  Kq_right_8/4(interp_point_4) -> n-D Lookup Table95/4
  Mux99/1 -> Product98/1
  n-D Lookup Table97/1 -> Mux90/1
  Constant121/1 -> Mux96/2
  Kq_left_out/3(interp_point_3) -> n-D Lookup Table88/3
  Kq_left_out/4(interp_point_4) -> n-D Lookup Table88/4
  Kq_tail_right/2(interp_point_2) -> n-D Lookup Table87/2
  Kq_right_10/3(interp_point_3) -> n-D Lookup Table97/3
  MATLAB Function192/1(Tail_Transform) -> Matrix Multiply80/1
  Matrix Multiply84/1 -> Add7/5
  Matrix Multiply95/1 -> Add7/10
  MATLAB Function98/1(Kq_Scale_5) -> Product84/2
  Constant117/1 -> Mux92/2
  MATLAB Function202/1(Wing_Transform) -> Matrix Multiply96/1
  MATLAB Function196/1(Wing_Transform) -> Matrix Multiply84/1
  MATLAB Function199/1(Wing_Transform) -> Matrix Multiply87/1
  MATLAB Function198/1(Wing_Transform) -> Matrix Multiply86/1
  Kq_left_6_in/4(interp_point_4) -> n-D Lookup Table93/4
  MATLAB Function194/1(Wing_Transform) -> Matrix Multiply82/1
  Product95/1 -> Matrix Multiply95/2
  MATLAB Function200/1(Wing_Transform) -> Matrix Multiply94/1
  Kq_right_12_out/1(interp_point_1) -> n-D Lookup Table99/1
  n-D Lookup Table95/1 -> Mux88/1
  MATLAB Function102/1(Kq_Scale_9) -> Product94/2
  n-D Lookup Table93/1 -> Mux97/1
  MATLAB Function203/1(Wing_Transform) -> Matrix Multiply97/1
  MATLAB Function96/1(Kq_Scale_3) -> Product74/2
  MATLAB Function197/1(Wing_Transform) -> Matrix Multiply85/1
  Kq_left_6_in/1(interp_point_1) -> n-D Lookup Table93/1
  Constant124/1 -> Mux100/2
  Add7/1 -> Out1/1
  Kq_right_9/4(interp_point_4) -> n-D Lookup Table96/4
  Mux90/1 -> Product97/1
